simulink model "VehicleModel"  (R2019b)
settings: Solver=VariableStepAuto  StartTime=0.0  StopTime=100  RelTol=1e-3
libraries: vrlib x3, simulink x1, mpcadaslib x1
settings Model: Creator=Yinglongli  LastModifiedBy=Yinglongli

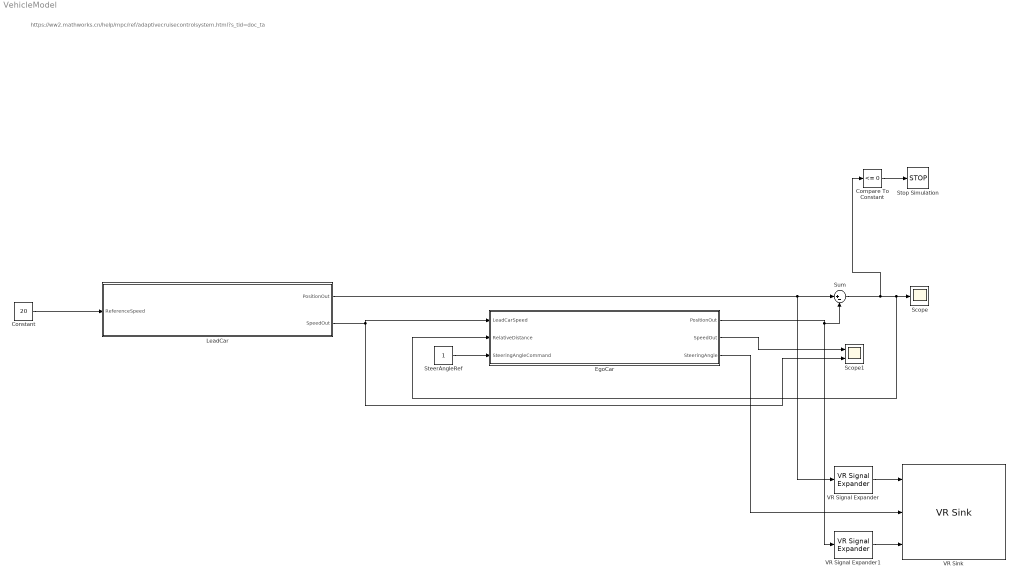
== system VehicleModel ==
  note: https://ww2.mathworks.cn/help/mpc/ref/adaptivecruisecontrolsystem.html?s_tid=doc_ta
  Compare To Constant : simulink/Logic and Bit Operations/Compare To Constant  relop=<=  const=0  OutDataTypeStr=boolean
  Constant : Constant  Value=20
  EgoCar : Subsystem  mask{InitialPos=0, InitialSpd=30}
      mask prompts: InitialPos "Initial Position"; InitialSpd "Initial Speed"
      mask TypeOptions InitialPos: InitialPos/Value
      mask TypeOptions InitialSpd: InitialSpd/Value
  LeadCar : Subsystem  mask{InitialPos=100, InitialSpd=20}
      mask prompts: InitialPos "Initial Position"; InitialSpd "Initial Speed"
      mask TypeOptions InitialPos: InitialPos/Value
      mask TypeOptions InitialSpd: InitialSpd/Value
  Scope : Scope
  Scope1 : Scope  NumInputPorts=2
  SteerAngleRef : Constant
  Stop Simulation : Stop
  Sum : Sum  Inputs=|+-
  VR Signal Expander : vrlib/VR Signal Expander  outwidth=3  outidx=[3]
      settings: SourceProductName=Simulink
  VR Signal Expander1 : vrlib/VR Signal Expander  outwidth=3  outidx=[3]
      settings: SourceProductName=Simulink
  VR Sink : vrlib/VR Sink  InstantiateOnLoad=on  SampleTime=0.02  ViewEnable=on  RemoteChange=off  RemoteView=off  FieldsWritten=Car_Red.translation.3.1.1.double#Car_Blue.rotation.4.1.1.double#Car_Blue.translation.3.1.1.double  WorldFileName=PlatoonWorld.WRL  AutoView=off  VideoDimensions=[]  AllowVariableSize=off
      settings: SourceProductName=Simulink
  wires:
  Constant/1 -> LeadCar/1(ReferenceSpeed)
  LeadCar/1(PositionOut) -> VR Signal Expander/1, Sum/1
  EgoCar/1(PositionOut) -> VR Signal Expander1/1, Sum/2
  EgoCar/2(SpeedOut) -> Scope1/1
  LeadCar/2(SpeedOut) -> EgoCar/1(LeadCarSpeed), Scope1/2
  Sum/1 -> Compare To Constant/1, EgoCar/2(RelativeDistance), Scope/1
  Compare To Constant/1 -> Stop Simulation/1
  SteerAngleRef/1 -> EgoCar/3(SteeringAngleCommand)
  VR Signal Expander/1 -> VR Sink/1
  VR Signal Expander1/1 -> VR Sink/3
  EgoCar/3(SteeringAngle) -> VR Sink/2

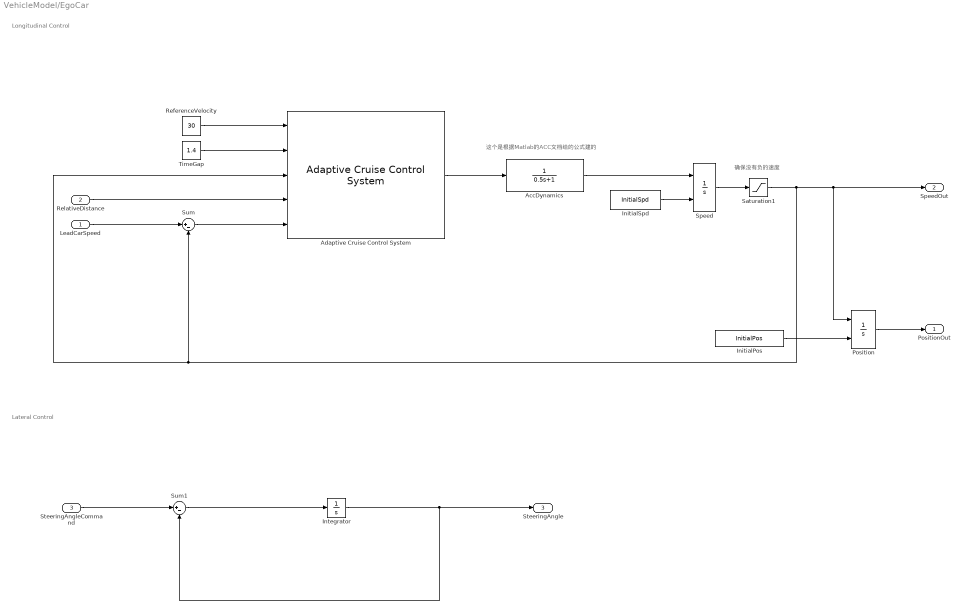
== system VehicleModel/EgoCar ==
  note: Longitudinal Control
  note: 确保没有负的速度
  note: 这个是根据Matlab的ACC文档给的公式建的
  note: Lateral Control
  LeadCarSpeed : Inport
  RelativeDistance : Inport  Port=2
  SteeringAngleCommand : Inport  Port=3
  AccDynamics : TransferFcn  Denominator=[0.5 1]
  Adaptive Cruise Control System : mpcadaslib/Adaptive Cruise Control System  EgoModel=tf(1,[0.5,1,0])  InitialEgoVelocity=20  DefaultSpacing=10  MaxVelocity=50  MinAcceleration=-3  amin_ext=off  MaxAcceleration=2  amax_ext=off  Ts=0.1  PredictionHorizon=200  ControllerBehavior=0.5  suboptimal=off  maxiter=10  datatypeopt=double  optmode=off  trackmode=off
      settings: SourceProductName=Model Predictive Control Toolbox
  InitialPos : Constant  Value=InitialPos
  InitialSpd : Constant  Value=InitialSpd
  Integrator : Integrator
  Position : Integrator  InitialConditionSource=external
  ReferenceVelocity : Constant  Value=30
  Saturation1 : Saturate  UpperLimit=inf  LowerLimit=0
  Speed : Integrator  InitialConditionSource=external
  Sum : Sum  Inputs=|+-
  Sum1 : Sum  Inputs=|+-
  TimeGap : Constant  Value=1.4
  PositionOut : Outport
  SpeedOut : Outport  Port=2
  SteeringAngle : Outport  Port=3
  wires:
  AccDynamics/1 -> Speed/1
  Saturation1/1 -> SpeedOut/1, Position/1, Adaptive Cruise Control System/3, Sum/2
  Speed/1 -> Saturation1/1
  LeadCarSpeed/1 -> Sum/1
  Sum/1 -> Adaptive Cruise Control System/5
  InitialSpd/1 -> Speed/2
  InitialPos/1 -> Position/2
  Adaptive Cruise Control System/1 -> AccDynamics/1
  Position/1 -> PositionOut/1
  RelativeDistance/1 -> Adaptive Cruise Control System/4
  TimeGap/1 -> Adaptive Cruise Control System/2
  ReferenceVelocity/1 -> Adaptive Cruise Control System/1
  SteeringAngleCommand/1 -> Sum1/1
  Sum1/1 -> Integrator/1
  Integrator/1 -> Sum1/2, SteeringAngle/1

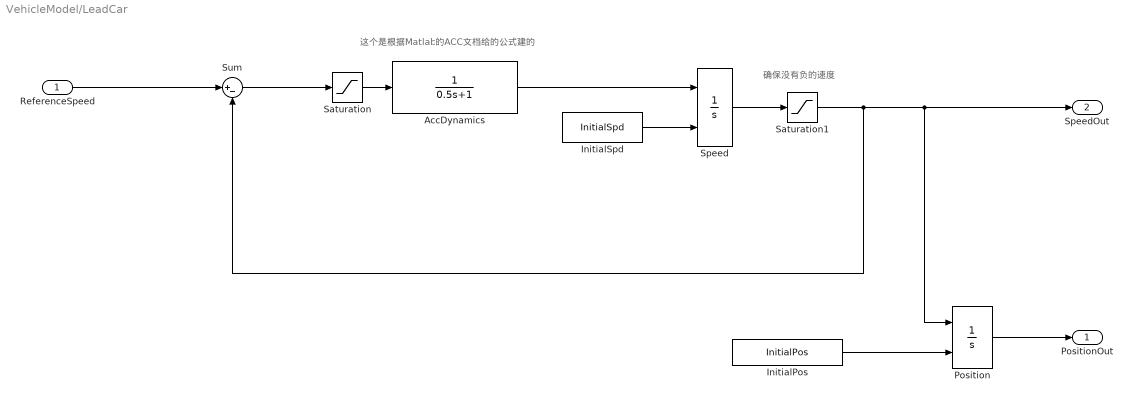
== system VehicleModel/LeadCar ==
  note: 确保没有负的速度
  note: 这个是根据Matlab的ACC文档给的公式建的
  ReferenceSpeed : Inport
  AccDynamics : TransferFcn  Denominator=[0.5 1]
  InitialPos : Constant  Value=InitialPos
  InitialSpd : Constant  Value=InitialSpd
  Position : Integrator  InitialConditionSource=external
  Saturation : Saturate  UpperLimit=2  LowerLimit=-3
  Saturation1 : Saturate  UpperLimit=inf  LowerLimit=0
  Speed : Integrator  InitialConditionSource=external
  Sum : Sum  Inputs=|+-
  PositionOut : Outport
  SpeedOut : Outport  Port=2
  wires:
  AccDynamics/1 -> Speed/1
  Saturation1/1 -> SpeedOut/1, Position/1, Sum/2
  Speed/1 -> Saturation1/1
  ReferenceSpeed/1 -> Sum/1
  Sum/1 -> Saturation/1
  InitialSpd/1 -> Speed/2
  InitialPos/1 -> Position/2
  Saturation/1 -> AccDynamics/1
  Position/1 -> PositionOut/1
